simulink model "ACC_detailed_model"  (R2018a)
settings: Solver=VariableStepAuto  StartTime=0.0  StopTime=250  RelTol=1e-3
InitFcn:
  | Jw = 4.5; % Inertia Kg.m^2
  | r = 0.3; % Radius of Wheel
  | Cf = 0.1; % Viscous coefficient
  | 
  | r=0.3; % Radius of wheel
  |  %Dry Asphalt road%
  | C1 = 1.2801;
  | C2 = 23.99;
  | C3 = 0.52;
  | 
  | M = 1300; % 1500Kg
  | g = 9.81; % m/s2
  | Cr = 0.01;				% coefficient of rolling friction
  | rho = 1.3;				% density of air, kg/m^3
  | Cd = 0.46;				% drag coefficient
libraries: simulink x1
settings Model: Creator=CHIZOM WORNU  LastModifiedBy=CHIZOM WORNU

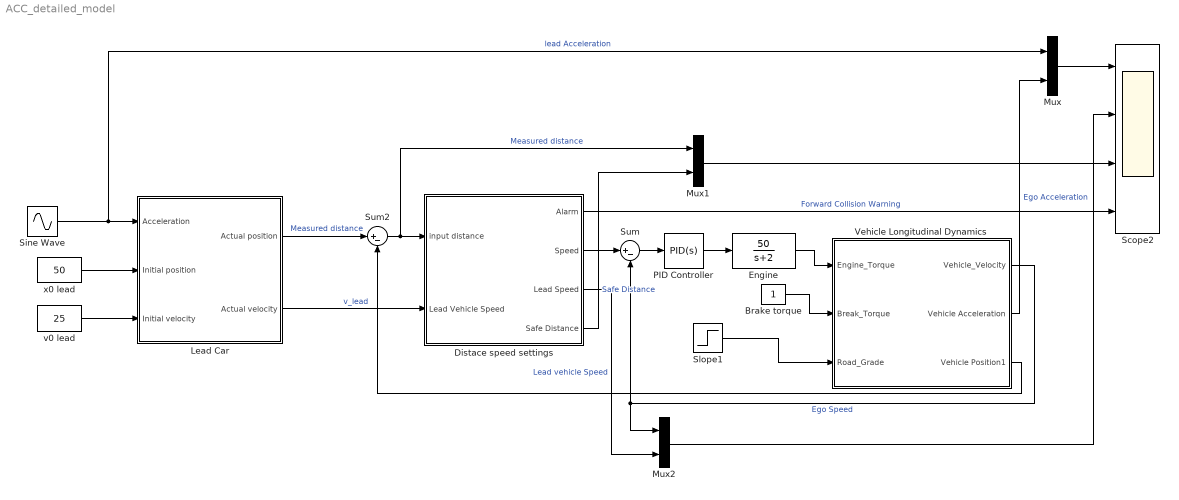
== system ACC_detailed_model ==
  Brake torque : Constant
  Distace speed settings : Subsystem
  Engine : TransferFcn  Numerator=50  Denominator=[1 2]
  Lead Car : Subsystem
  Mux : Mux  Inputs=2
  Mux1 : Mux  Inputs=2
  Mux2 : Mux  Inputs=2
  PID Controller : simulink/Continuous/PID Controller  Controller=PID  TimeDomain=Continuous-time  SampleTime=-1  IntegratorMethod=Forward Euler  FilterMethod=Forward Euler  Form=Parallel  UseFilter=on  ControllerParametersSource=internal  P=30.0096454190468  I=4.39323599940394  D=-0.171141386307986  N=175.350019457254  InitialConditionSource=internal  InitialConditionForIntegrator=0  InitialConditionForFilter=0  ExternalReset=none  LimitOutput=off  UpperSaturationLimit=inf  LowerSaturationLimit=-inf  LinearizeAsGain=on  AntiWindupMode=none  Kb=1  TrackingMode=off  Kt=1  PParamMin=[]  PParamMax=[]  IParamMin=[]  IParamMax=[]  DParamMin=[]  DParamMax=[]  NParamMin=[]  NParamMax=[]  KbParamMin=[]  KbParamMax=[]  KtParamMin=[]  KtParamMax=[]  POutMin=[]  POutMax=[]  IOutMin=[]  IOutMax=[]  DOutMin=[]  DOutMax=[]  NOutMin=[]  NOutMax=[]  KbOutMin=[]  KbOutMax=[]  KtOutMin=[]  KtOutMax=[]  IntegratorOutMin=[]  IntegratorOutMax=[]  FilterOutMin=[]  FilterOutMax=[]  SumOutMin=[]  SumOutMax=[]  SumI1OutMin=[]  SumI1OutMax=[]  SumI2OutMin=[]  SumI2OutMax=[]  SumI3OutMin=[]  SumI3OutMax=[]  SumDOutMin=[]  SumDOutMax=[]  SaturationOutMin=[]  SaturationOutMax=[]  IntegratorContinuousStateAttributes=''  IntegratorStateMustResolveToSignalObject=off  IntegratorRTWStateStorageClass=Auto  FilterContinuousStateAttributes=''  FilterStateMustResolveToSignalObject=off  FilterRTWStateStorageClass=Auto  DifferentiatorICPrevScaledInput=0  DifferentiatorOutMin=[]  DifferentiatorOutMax=[]  InitialConditionSetting=State (most efficient)  FilterDiffOutCoefMin=[]  FilterDiffOutCoefMax=[]  SumDenOutMin=[]  SumDenOutMax=[]  SumNumOutMin=[]  SumNumOutMax=[]  ReciprocalOutMin=[]  ReciprocalOutMax=[]  DivideOutMin=[]  DivideOutMax=[]  TunerSelectOption=Transfer Function Based (PID Tuner App)
  Scope2 : Scope  NumInputPorts=4
  Sine Wave : Sin  Amplitude=0.5  Frequency=0.2  SampleTime=0.1
  Slope1 : Step  Time=50  After=0  SampleTime=0
  Sum : Sum  Inputs=|+-
  Sum2 : Sum  Inputs=|+-
  Vehicle Longitudinal Dynamics : Subsystem
  v0 lead : Constant  Value=25  SampleTime=0.1
  x0 lead : Constant  Value=50  SampleTime=0.1
  wires:
  Vehicle Longitudinal Dynamics/1(Vehicle_Velocity) -> Mux2/1, Sum/2  "Ego Speed"
  Mux/1 -> Scope2/1
  Distace speed settings/3(Lead Speed) -> Mux2/2  "Lead vehicle Speed"
  Brake torque/1 -> Vehicle Longitudinal Dynamics/2(Break_Torque)
  Distace speed settings/1(Alarm) -> Scope2/4  "Forward Collision Warning"
  Sum/1 -> PID Controller/1
  Distace speed settings/2(Speed) -> Sum/1
  Slope1/1 -> Vehicle Longitudinal Dynamics/3(Road_Grade)
  PID Controller/1 -> Engine/1
  Engine/1 -> Vehicle Longitudinal Dynamics/1(Engine_Torque)
  Sum2/1 -> Distace speed settings/1(input distance), Mux1/1  "Measured distance"
  Lead Car/2(Actual velocity) -> Distace speed settings/2(Lead Vehicle Speed)  "v_lead"
  x0 lead/1 -> Lead Car/2(Initial position)
  v0 lead/1 -> Lead Car/3(Initial velocity)
  Sine Wave/1 -> Mux/1, Lead Car/1(Acceleration)  "lead Acceleration"
  Lead Car/1(Actual position) -> Sum2/1  "Measured distance"
  Vehicle Longitudinal Dynamics/3(Vehicle Position1) -> Sum2/2
  Distace speed settings/4(Safe Distance) -> Mux1/2  "Safe Distance"
  Mux2/1 -> Scope2/2
  Mux1/1 -> Scope2/3
  Vehicle Longitudinal Dynamics/2(Vehicle Acceleration) -> Mux/2  "Ego Acceleration"

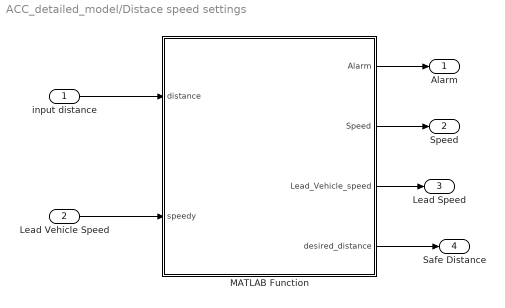
== system ACC_detailed_model/Distace speed settings ==
  input distance : Inport
  Lead Vehicle Speed : Inport  Port=2
  MATLAB Function : MATLAB Function  TreatAsAtomicUnit=on
  Alarm : Outport
  Speed : Outport  Port=2
  Lead Speed : Outport  Port=3
  Safe Distance : Outport  Port=4
  wires:
  MATLAB Function/1(Alarm) -> Alarm/1
  input distance/1 -> MATLAB Function/1(distance)
  MATLAB Function/3(Lead_Vehicle_speed) -> Lead Speed/1
  MATLAB Function/2(Speed) -> Speed/1
  Lead Vehicle Speed/1 -> MATLAB Function/2(speedy)
  MATLAB Function/4(desired_distance) -> Safe Distance/1

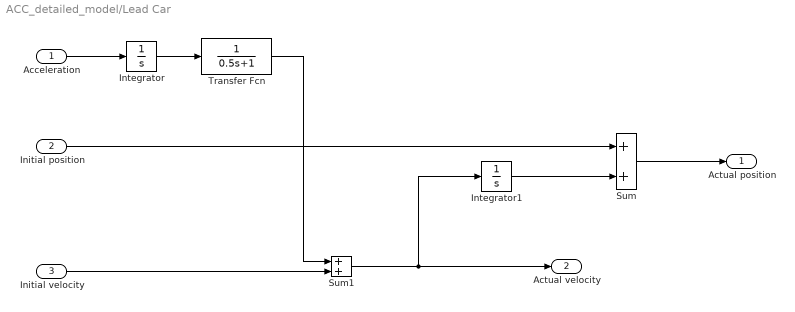
== system ACC_detailed_model/Lead Car ==
  Acceleration : Inport
  Initial position : Inport  Port=2
  Initial velocity : Inport  Port=3
  Integrator : Integrator
  Integrator1 : Integrator
  Sum : Sum
  Sum1 : Sum
  Transfer Fcn : TransferFcn  Denominator=[0.5 1]
  Actual position : Outport
  Actual velocity : Outport  Port=2
  wires:
  Transfer Fcn/1 -> Sum1/1
  Initial velocity/1 -> Sum1/2
  Sum/1 -> Actual position/1
  Integrator/1 -> Transfer Fcn/1
  Sum1/1 -> Integrator1/1, Actual velocity/1
  Acceleration/1 -> Integrator/1
  Initial position/1 -> Sum/1
  Integrator1/1 -> Sum/2

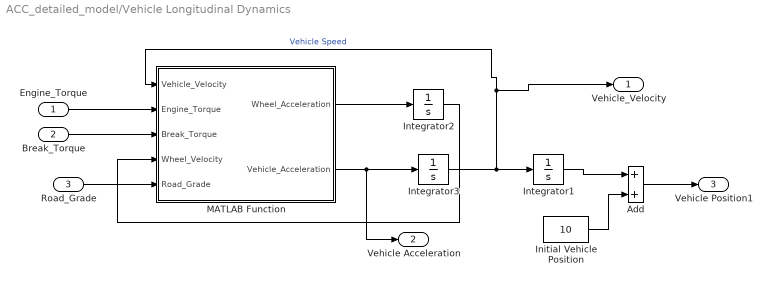
== system ACC_detailed_model/Vehicle Longitudinal Dynamics ==
  Engine_Torque : Inport
  Break_Torque : Inport  Port=2
  Road_Grade : Inport  Port=3
  Add : Sum
  Initial Vehicle Position : Constant  Value=10  SampleTime=0.1
  Integrator1 : Integrator  InitialCondition=1
  Integrator2 : Integrator  InitialCondition=1
  Integrator3 : Integrator  InitialCondition=1
  MATLAB Function : MATLAB Function  TreatAsAtomicUnit=on
  Vehicle_Velocity : Outport
  Vehicle Acceleration : Outport  Port=2
  Vehicle Position1 : Outport  Port=3
  wires:
  MATLAB Function/1(Wheel_Acceleration) -> Integrator2/1
  Integrator2/1 -> MATLAB Function/4(Wheel_Velocity)
  MATLAB Function/2(Vehicle_Acceleration) -> Vehicle Acceleration/1, Integrator3/1
  Integrator3/1 -> Vehicle_Velocity/1, MATLAB Function/1(Vehicle_Velocity), Integrator1/1  "Vehicle Speed"
  Integrator1/1 -> Add/1
  Initial Vehicle Position/1 -> Add/2
  Add/1 -> Vehicle Position1/1
  Road_Grade/1 -> MATLAB Function/5(Road_Grade)
  Break_Torque/1 -> MATLAB Function/3(Break_Torque)
  Engine_Torque/1 -> MATLAB Function/2(Engine_Torque)

== matlab function ACC_detailed_model/Vehicle Longitudinal Dynamics/MATLAB Function ==
  data: Vehicle_Velocity input; Engine_Torque input; Wheel_Acceleration output; Break_Torque input; Wheel_Velocity input; Vehicle_Acceleration output; Road_Grade input
function [Wheel_Acceleration,Vehicle_Acceleration]  = fcn(Vehicle_Velocity,Engine_Torque, Break_Torque, Wheel_Velocity, Road_Grade)

Jw = 4.5; % Inertia Kg.m^2
%r = 0.3; % Radius of Wheel
Cf = 0.1; % Viscous coefficient

r=0.3; % Radius of wheel
 %Dry Asphalt road%
C1 = 1.2801;
C2 = 23.99;
C3 = 0.52;

M = 1300; % 1500Kg
g = 9.81; % m/s2
Cr = 0.01;				% coefficient of rolling friction
rho = 1.3;				% density of air, kg/m^3
Cd = 0.46;				% drag coefficient

Slip = (Vehicle_Velocity-(r*Wheel_Velocity))/Vehicle_Velocity; %Slip equation
u = C1-(C1*exp(-C2*Slip))-C3*Slip; % Equation of friction

A = 1.6 + 0.00056*(M-765);				% car area, m^2

Fr = M * g * Cr	;		% Rolling friction
Fa = 0.5 * rho * Cd * A * Vehicle_Velocity*Vehicle_Velocity;		% Aerodynamic drag
Fg = M * g * sin(Road_Grade);		% Road slope force
Fd = Fr + Fa + Fg;			% total deceleration
Fz = M * g * cos(Road_Grade); % Normal Force
Fx = 4*u*Fz; % Driving Force

Wheel_Acceleration = (Engine_Torque-Break_Torque-Wheel_Velocity*Cf-r*Fx)/Jw; % Wheel acceleration
Vehicle_Acceleration = (Fx-Fd)/M; % Acceleration of the vehicle

== matlab function ACC_detailed_model/Distace speed settings/MATLAB Function ==
  data: distance input; Alarm output; Speed output; Lead_Vehicle_speed output; speedy input; desired_distance output
function [Alarm, Speed,Lead_Vehicle_speed,desired_distance] = fcn(distance,speedy)
maxspeed=30;
Alarm1=0;  %Initializing the Alarm
speed1=0;  %Initializing the speed
Default_Spacing_distance = 5; % Default Safe distance between both vehicles
THW= 1.5; %Time Headway
desired_distance = Default_Spacing_distance + speedy*THW; % Desired Distance or safe distance
error_distance=distance-desired_distance; % Distance Error
% speedy is the vehicles speed feed back into the system
Lead_Vehicle_speed = (speedy + (error_distance*0.1)); % Lead vehicles Speed
min_distance = 2; % Minimum Distance

% Constrain 1
if distance >= desired_distance
    speed1 = maxspeed;
    % Constrain 2
elseif distance <= 3%min_distance
    speed1 = 0;
end
% Constrain 3
if distance <  desired_distance && distance >= min_distance
    if Lead_Vehicle_speed>maxspeed
        speed1 = maxspeed;
    else
        speed1 = Lead_Vehicle_speed+0.01;
    end
end
%Distance Alert and Forward Collsion Warning
% Constrain 4
if distance <= 40 && distance >20
    Alarm1 = 25; %Distance Alert
    % Constrain 5
elseif distance > min_distance && distance <=20
    Alarm1 = 50; %Forward Collsion Warning
end

Alarm=Alarm1;
Speed=speed1;
